simulink model "Punto_5b"  (R2023a)
settings: Solver=VariableStepAuto  StartTime=0.0  StopTime=20  RelTol=1e-3
libraries: simulink x2
settings Model: Creator=garzo  LastModifiedBy=laura
settings ModelReferenceCC: EnableRefExpFcnMdlSchedulingChecks=on

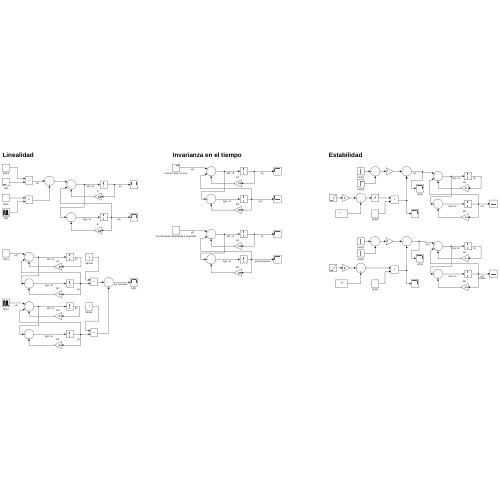
[thumbnail: Simulink's stored preview of the top-level diagram]
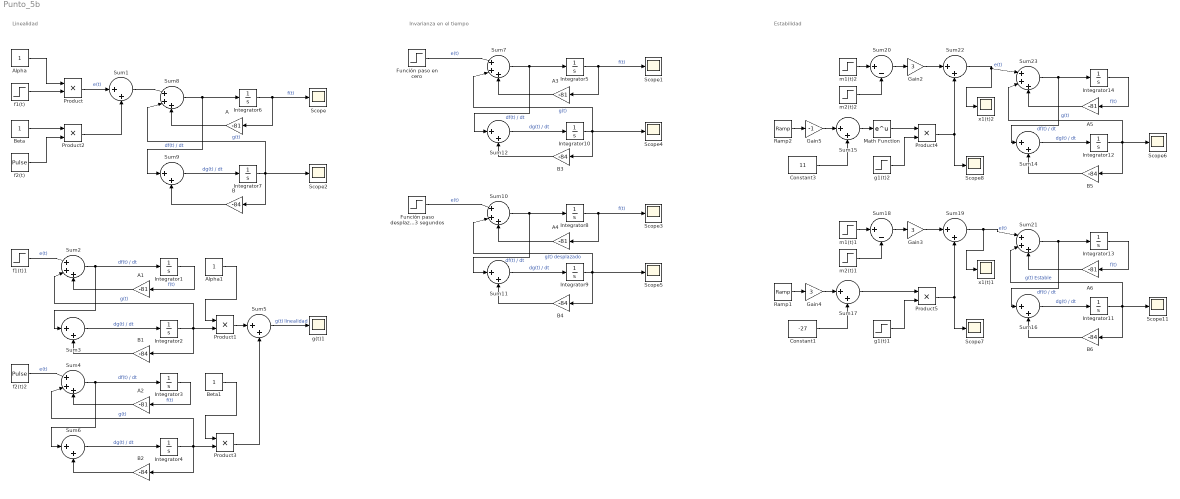
== system Punto_5b ==
  note: Linealidad
  note: Invarianza en el tiempo
  note: Estabilidad
  A{,1..6} (7 alike) : Gain  Gain=-81
  Alpha : Constant
  Alpha1 : Constant
  B{,1..6} (7 alike) : Gain  Gain=-84
  Beta : Constant
  Beta1 : Constant
  Constant1 : Constant  Value=-27
  Constant3 : Constant  Value=11
  Función paso desplazada 3 segundos : Step  Time=5  SampleTime=0
  Función paso en cero : Step  Time=0  SampleTime=0
  Gain2 : Gain  Gain=3
  Gain3 : Gain  Gain=3
  Gain4 : Gain  Gain=3
  Gain5 : Gain  Gain=-1
  Integrator{1..14} (14 alike) : Integrator
  Math Function : Math
  Product{,1..5} (6 alike) : Product
  Ramp1 : simulink/Sources/Ramp  slope=1  start=0  InitialOutput=0
  Ramp2 : simulink/Sources/Ramp  slope=1  start=0  InitialOutput=0
  Scope{,1..8,11} (10 alike) : Scope
  Sum{1,3,5..6,9,11..12,14..17,19,22} (13 alike) : Sum  Inputs=|++
  Sum{2,4,7..8,10,21,23} (7 alike) : Sum  Inputs=|+++
  Sum18 : Sum  Inputs=|+-
  Sum20 : Sum  Inputs=|+-
  f1(t) : Step  SampleTime=0
  f1(t)1 : Step  SampleTime=0
  f2(t) : DiscretePulseGenerator  PulseType=Time based  Period=10  PulseWidth=5
  f2(t)2 : DiscretePulseGenerator  PulseType=Time based  Period=10  PulseWidth=5
  g(t)1 : Scope
  g1(t)1 : Step  Time=10  SampleTime=0
  g1(t)2 : Step  Time=10  SampleTime=0
  m1(t)1 : Step  Time=0  SampleTime=0
  m1(t)2 : Step  Time=0  SampleTime=0
  m2(t)1 : Step  Time=10  SampleTime=0
  m2(t)2 : Step  Time=10  SampleTime=0
  x1(t)1 : Scope
  x1(t)2 : Scope
  wires:
  Alpha/1 -> Product/1
  f1(t)/1 -> Product/2
  f2(t)/1 -> Product2/2
  Product2/1 -> Sum1/2
  Product/1 -> Sum1/1  "e(t)"
  Beta/1 -> Product2/1
  Product1/1 -> Sum5/1
  Beta1/1 -> Product3/1
  Product3/1 -> Sum5/2
  Alpha1/1 -> Product1/1
  Sum5/1 -> g(t)1/1  "g(t) linealidad"
  Sum8/1 -> Sum9/1, Integrator6/1  "df(t) / dt"
  A/1 -> Sum8/3
  Integrator7/1 -> B/1, Scope2/1, Sum8/2  "g(t)"
  Sum1/1 -> Sum8/1
  Integrator6/1 -> A/1, Scope/1  "f(t)"
  Sum9/1 -> Integrator7/1  "dg(t) / dt"
  B/1 -> Sum9/2
  Integrator2/1 -> B1/1, Product1/2, Sum2/2  "g(t)"
  B1/1 -> Sum3/2
  Sum3/1 -> Integrator2/1  "dg(t) / dt"
  Integrator1/1 -> A1/1  "f(t)"
  f1(t)1/1 -> Sum2/1  "e(t)"
  Sum2/1 -> Sum3/1, Integrator1/1  "df(t) / dt"
  A1/1 -> Sum2/3
  Integrator4/1 -> B2/1, Product3/2, Sum4/2  "g(t)"
  Integrator3/1 -> A2/1  "f(t)"
  Sum4/1 -> Sum6/1, Integrator3/1  "df(t) / dt"
  Sum6/1 -> Integrator4/1  "dg(t) / dt"
  A2/1 -> Sum4/3
  B2/1 -> Sum6/2
  f2(t)2/1 -> Sum4/1  "e(t)"
  Integrator10/1 -> B3/1, Scope4/1, Sum7/2  "g(t)"
  B3/1 -> Sum12/2
  Sum12/1 -> Integrator10/1  "dg(t) / dt"
  Integrator5/1 -> A3/1, Scope1/1  "f(t)"
  Función paso en cero/1 -> Sum7/1  "e(t)"
  Sum7/1 -> Sum12/1, Integrator5/1  "df(t) / dt"
  A3/1 -> Sum7/3
  Integrator9/1 -> B4/1, Scope5/1, Sum10/2  "g(t) desplazado"
  B4/1 -> Sum11/2
  Sum11/1 -> Integrator9/1  "dg(t) / dt"
  Integrator8/1 -> A4/1, Scope3/1  "f(t)"
  Función paso desplazada 3 segundos/1 -> Sum10/1  "e(t)"
  Sum10/1 -> Sum11/1, Integrator8/1  "df(t) / dt"
  A4/1 -> Sum10/3
  Ramp1/1 -> Gain4/1
  Sum17/1 -> Product5/1
  g1(t)1/1 -> Product5/2
  Gain4/1 -> Sum17/1
  m2(t)1/1 -> Sum18/2
  m1(t)1/1 -> Sum18/1
  Sum18/1 -> Gain3/1
  Gain3/1 -> Sum19/1
  Product5/1 -> Scope7/1, Sum19/2
  Constant1/1 -> Sum17/2
  Integrator13/1 -> A6/1  "f(t)"
  Sum19/1 -> x1(t)1/1, Sum21/1  "e(t)"
  A6/1 -> Sum21/3
  Integrator11/1 -> Sum21/2, Scope11/1, B6/1  "g(t) Estable"
  Sum21/1 -> Integrator13/1, Sum16/1  "df(t) / dt"
  B6/1 -> Sum16/2
  Sum16/1 -> Integrator11/1  "dg(t) / dt"
  Sum14/1 -> Integrator12/1  "dg(t) / dt"
  Gain5/1 -> Sum15/1
  Product4/1 -> Scope8/1, Sum22/2
  Integrator14/1 -> A5/1  "f(t)"
  Constant3/1 -> Sum15/2
  Sum20/1 -> Gain2/1
  g1(t)2/1 -> Product4/2
  Sum23/1 -> Integrator14/1, Sum14/1  "df(t) / dt"
  m2(t)2/1 -> Sum20/2
  Gain2/1 -> Sum22/1
  Integrator12/1 -> Sum23/2, Scope6/1, B5/1  "g(t)"
  Ramp2/1 -> Gain5/1
  m1(t)2/1 -> Sum20/1
  B5/1 -> Sum14/2
  A5/1 -> Sum23/3
  Sum15/1 -> Math Function/1
  Math Function/1 -> Product4/1
  Sum22/1 -> x1(t)2/1, Sum23/1  "e(t)"
